simulink model "full_automaton2017a"  (R2017a)
settings: Solver=VariableStepAuto  StartTime=0.0  StopTime=10.0  RelTol=1e-3
settings Model: Creator=gonzalo  LastModifiedBy=gonzalo

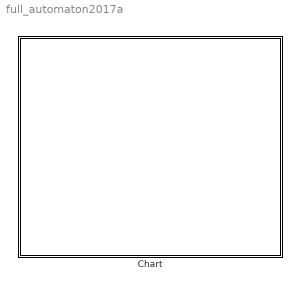
== system full_automaton2017a ==
  Chart : Stateflow chart  TreatAsAtomicUnit=on

== stateflow chart full_automaton2017a/Chart ==
  state Automaton
    state Level1 [parallel]
      settings: executionOrder=1
      state Start [parallel]
        settings: executionOrder=1
        state Manual
          entry:
          during:
        state Automatico
          entry:
          during:
        (default) -> Manual
        Manual -> Automatico : [automatic == 1]
        Automatico -> Manual : [automatic == 0]
      state Spreader [parallel]
        settings: executionOrder=2
        state Charged
        state Unchaged
        (default) -> Charged
        Charged -> Unchaged : [twistlocks == 0]
        Unchaged -> Charged : [twistlocks == 1]
      state Balancing_Control [parallel]
        settings: executionOrder=3
        state Activated
        state Disactivated
        (default) -> Activated
        Activated -> Disactivated : [balacing_control == 0]
        Disactivated -> Activated : [balancing_control == 1]
    state Level_0 [parallel]
      settings: executionOrder=2
      state Emergency_limit_switch_horizontal
        entry:
        emergency = 1;
        if (bottom_limit == 1)
        error = 1;
        else
        error = 2;
        end
      state Normal
        entry:
        emergency = 0;
        error = 0;
      state Emergency_limit_switch_vertical
        entry:
        emergency = 1;
        if (bottom_limit == 1)
        error = 3;
        else
        error = 4;
        end
      state Emergency_overspeed
        entry:
        emergency = 1;
        error = 5;
      state Emergency_button
        entry:
        emergency = 1;
        error = 6;
      Normal -> Emergency_limit_switch_horizontal [order 1] : [(right_limit == 1)||(left_limit == 1)]
      Normal -> Emergency_limit_switch_vertical [order 2] : [(top_limit == 1) || (bottom_limit == 1)]
      (default) -> Normal
      Normal -> Emergency_overspeed [order 4] : [overspeed == 1]
      Normal -> Emergency_button [order 3] : [push_button == 1]
  state Emergency
    state emergency_handler
      during:
      %emergency_routine()
    state end_emergency
      entry:
      emergency = 0
    (default) -> emergency_handler
    emergency_handler -> end_emergency : [error_fixed == 1]
  (default) -> Automaton
  Automaton -> Emergency : [emergency == 1]
  Emergency -> Automaton : [emergency == 0]
